simulink library "dynamicPressure_ul"  (R2018b)
settings: Solver=VariableStepAuto  StartTime=0.0  StopTime=10.0  RelTol=1e-3
settings Model: Creator=asiddiq2  LastModifiedBy=asiddiq2

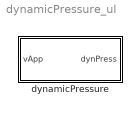
== system dynamicPressure_ul ==
  dynamicPressure : Subsystem  mask{rhoFluid=0}
      mask prompts: rhoFluid "Fluid density"

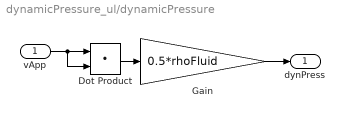
== system dynamicPressure_ul/dynamicPressure ==
  vApp : Inport
  Dot Product : DotProduct  InputSameDT=on  OutDataTypeStr=Inherit: Inherit via internal rule
  Gain : Gain  Gain=0.5*rhoFluid
  dynPress : Outport
  wires:
  vApp/1 -> Dot Product/2, Dot Product/1
  Dot Product/1 -> Gain/1
  Gain/1 -> dynPress/1
